simulink model "gridguard_model"  (R2026a)
settings: Solver=ode4  StopTime=30.0  FixedStep=0.01
settings Model: Creator=Ananya Tripathi  LastModifiedBy=Ananya Tripathi
settings DataIOCC: SignalLoggingName=logsOut

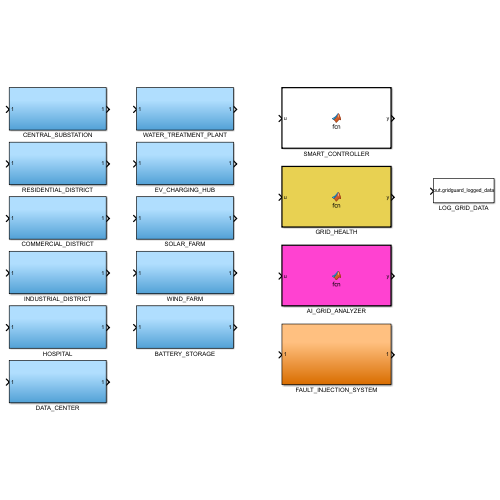
[thumbnail: Simulink's stored preview of the top-level diagram]
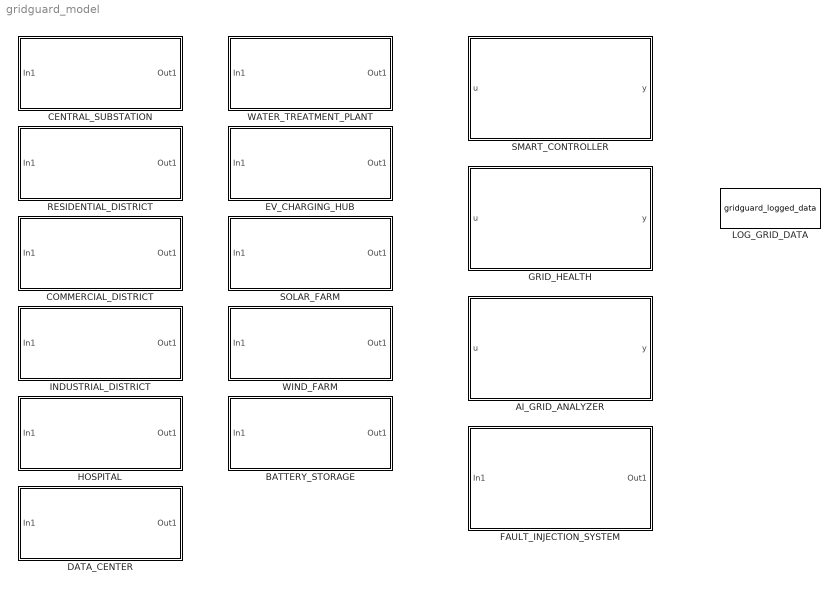
== system gridguard_model ==
  AI_GRID_ANALYZER : MATLAB Function  TreatAsAtomicUnit=on
  BATTERY_STORAGE : Subsystem
  CENTRAL_SUBSTATION : Subsystem
  COMMERCIAL_DISTRICT : Subsystem
  DATA_CENTER : Subsystem
  EV_CHARGING_HUB : Subsystem
  FAULT_INJECTION_SYSTEM : Subsystem
  GRID_HEALTH : MATLAB Function  TreatAsAtomicUnit=on
  HOSPITAL : Subsystem
  INDUSTRIAL_DISTRICT : Subsystem
  LOG_GRID_DATA : ToWorkspace  VariableName=gridguard_logged_data  SaveFormat=Timeseries  SampleTime=-1
  RESIDENTIAL_DISTRICT : Subsystem
  SMART_CONTROLLER : MATLAB Function  TreatAsAtomicUnit=on
  SOLAR_FARM : Subsystem
  WATER_TREATMENT_PLANT : Subsystem
  WIND_FARM : Subsystem

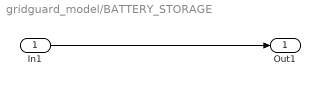
== system gridguard_model/BATTERY_STORAGE ==
  In1 : Inport
  Out1 : Outport
  wires:
  In1/1 -> Out1/1

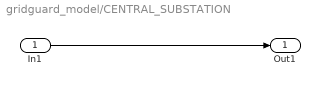
== system gridguard_model/CENTRAL_SUBSTATION ==
  In1 : Inport
  Out1 : Outport
  wires:
  In1/1 -> Out1/1

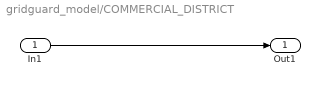
== system gridguard_model/COMMERCIAL_DISTRICT ==
  In1 : Inport
  Out1 : Outport
  wires:
  In1/1 -> Out1/1

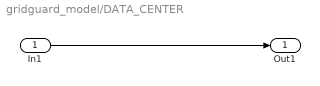
== system gridguard_model/DATA_CENTER ==
  In1 : Inport
  Out1 : Outport
  wires:
  In1/1 -> Out1/1

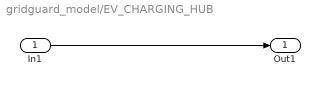
== system gridguard_model/EV_CHARGING_HUB ==
  In1 : Inport
  Out1 : Outport
  wires:
  In1/1 -> Out1/1

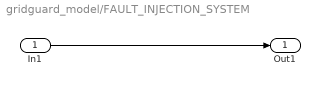
== system gridguard_model/FAULT_INJECTION_SYSTEM ==
  In1 : Inport
  Out1 : Outport
  wires:
  In1/1 -> Out1/1

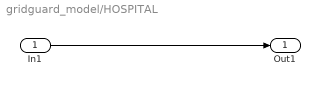
== system gridguard_model/HOSPITAL ==
  In1 : Inport
  Out1 : Outport
  wires:
  In1/1 -> Out1/1

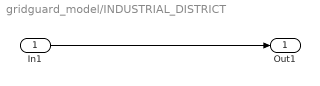
== system gridguard_model/INDUSTRIAL_DISTRICT ==
  In1 : Inport
  Out1 : Outport
  wires:
  In1/1 -> Out1/1

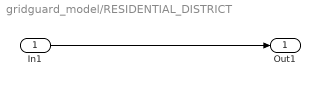
== system gridguard_model/RESIDENTIAL_DISTRICT ==
  In1 : Inport
  Out1 : Outport
  wires:
  In1/1 -> Out1/1

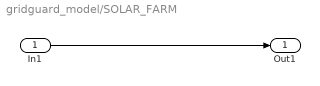
== system gridguard_model/SOLAR_FARM ==
  In1 : Inport
  Out1 : Outport
  wires:
  In1/1 -> Out1/1

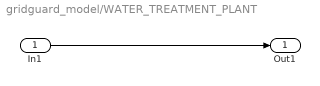
== system gridguard_model/WATER_TREATMENT_PLANT ==
  In1 : Inport
  Out1 : Outport
  wires:
  In1/1 -> Out1/1

== system gridguard_model/WIND_FARM ==
  In1 : Inport
  Out1 : Outport
  wires:
  In1/1 -> Out1/1

== matlab function gridguard_model/SMART_CONTROLLER ==
  data: u input; y output
function y = fcn(u)

y = u;

== matlab function gridguard_model/AI_GRID_ANALYZER ==
  data: u input; y output
function y = fcn(u)

y = u;

== matlab function gridguard_model/GRID_HEALTH ==
  data: u input; y output
function y = fcn(u)

y = u;
